simulink model "Controller_Exp"  (R2016a)
settings: Solver=ode4  StartTime=0.0  StopTime=Inf  FixedStep=Ts  RelTol=1e-3
undefined symbols (not defined in the file or in its folder): A_lpf_velocity, B1_lpf_velocity, B2_lpf_velocity, Calibration, commanded_u, GearOffsets, IMUTorsoOffsets, MedullaCommand, ResetDAQ, sample_time, TorsoCOMOffsets, Ts
libraries: xpcethercatlib x188, simulink x37, slrtlib x11, ControllerLibrary x2, dspswit3 x1
(part 1 of 4)
settings Model: TunableVars=GaitLibrary,GearOffsets,LegHipTorqueLimit,LimitSwHipAngle_ctrl,MedullaCommand,amp_ctrl,commanded_u,deltaStKA_ctrl,deltaSwHA_ctrl,deltaSwKA_ctrl,deltaSwLA_ctrl,floatDamper_ctrl,footPlacementHA_ctrl,footPlacementLA_ctrl,freq_ctrl,hold_ctrl,isTest_constantHips,isTest_doubleSupport,isTest_hipTracking,isTest_holdInAir,isTest_stopAndGo,jointPassivity_ctrl,joint_test_amp_ctrl,joint_test_freq_ctrl,joint_test_link_num_ctrl,joint_zero_ctrl,kd_ctrl,kd_hip_ctrl,kd_pitch,kd_roll,kd_sha,kd_sla,kd_stanceHip,kd_stanceKnee,kd_stanceLeg,kd_swingHip,kd_swingKnee,kd_swingLeg,kf_knee,kf_sha,kf_sla,kg_sha,kg_sla,ki_sha,ki_sla,kp_ctrl,kp_hip_ctrl,kp_pitch,kp_roll,kp_sha,kp_sla,kp_stanceHip,kp_stanceKnee,kp_stanceLeg,kp_swingHip,kp_swingKnee,kp_swingLeg,kp_yaw,leg_length,link_num_ctrl,ps3Axes,ps3Buttons,ps3Pov,regulate_velocity_ctrl,s_hold_ctrl,s_period_ctrl,stepTime,thres_hi,thres_lo,torso_com_offset,torso_control_ctrl,uHipGravity,zero_error_ctrl  TunableVarsStorageClass=Auto,Auto,Auto,Auto,Auto,Auto,Auto,Auto,Auto,Auto,Auto,Auto,Auto,Auto,Auto,Auto,Auto,Auto,Auto,Auto,Auto,Auto,Auto,Auto,Auto,Auto,Auto,Auto,Auto,Auto,Auto,Auto,Auto,Auto,Auto,Auto,Auto,Auto,Auto,Auto,Auto,Auto,Auto,Auto,Auto,Auto,Auto,Auto,Auto,Auto,Auto,Auto,Auto,Auto,Auto,Auto,Auto,Auto,Auto,Auto,Auto,Auto,Auto,Auto,Auto,Auto,Auto,Auto,Auto,Auto,Auto,Auto,Auto  TunableVarsTypeQualifier=,,,,,,,,,,,,,,,,,,,,,,,,,,,,,,,,,,,,,,,,,,,,,,,,,,,,,,,,,,,,,,,,,,,,,,,,  Creator=mvetsch  LastModifiedBy=gyk
settings SolverCC: EnableConcurrentExecution=on
settings DataIOCC: SaveFormat=Structure  SignalLoggingSaveFormat=ModelDataLogs  SaveState=on  SignalLoggingName=logsOut
settings OptimizationCC: BlockReduction=off  BooleanDataType=off  DefaultParameterBehavior=Inlined  OptimizeBlockIOStorage=off  BufferReuse=off  GlobalBufferReuse=off  ExpressionFolding=off  LocalBlockOutputs=off  InitFltsAndDblsToZero=on
settings DebuggingCC: SaveWithParameterizedLinksMsg=none  CheckExecutionContextPreStartOutputMsg=on  CheckExecutionContextRuntimeOutputMsg=on  SignalResolutionControl=TryResolveAllWithWarning  MultiTaskDSMMsg=warning  MultiTaskCondExecSysMsg=none
settings HardwareCC: ProdBitPerPointer=32  ProdLargestAtomicFloat=None  ProdWordSize=32  ProdLongLongMode=on  ProdHWDeviceType=Generic->32-bit x86 compatible
settings ModelReferenceCC: PropagateSignalLabelsOutOfModel=off
settings RTWCC: SystemTargetFile=slrt.tlc  TemplateMakefile=slrt_default_tmf  Description=Simulink Real-Time
settings SimulinkRealTimeCC: GeneratePreprocessorConditionals=Disable all  RL32LogBufSizeModifier=40000000  xPCisDownloadable=off
settings ConfigComp: CovModelRefEnable=Off  CovSFcnEnable=off

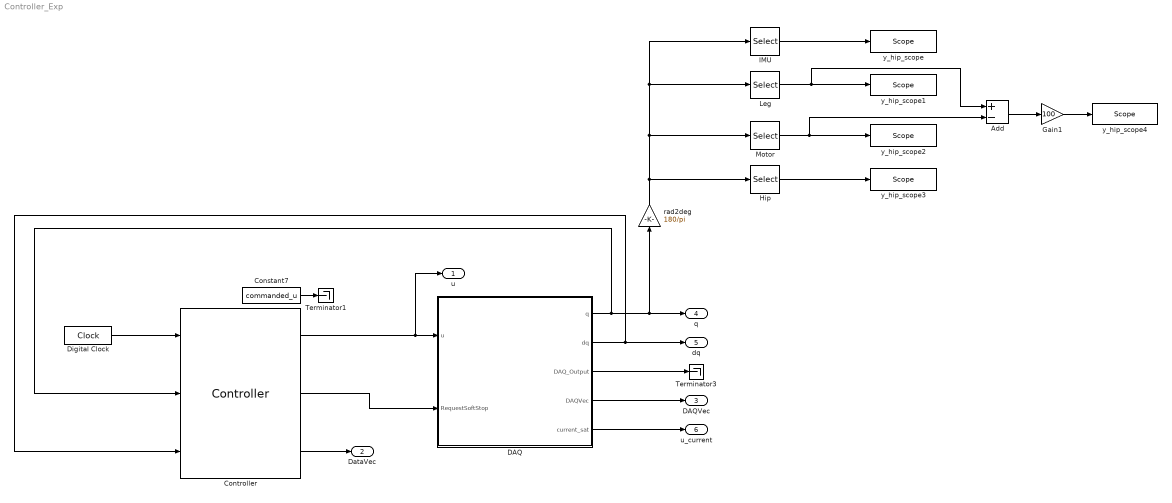
== system Controller_Exp ==
  Add : Sum  Inputs=+-
  Constant7 : Constant  Value=commanded_u
  Controller : ControllerLibrary/Controller
  DAQ : Subsystem
  Digital Clock : DigitalClock  SampleTime=Ts
  Gain1 : Gain  Gain=100
  Hip : Selector  InputPortWidth=13  IndexOptions=Index vector (dialog)  Indices=[10 13]  OutputSizes=1
  IMU : Selector  InputPortWidth=13  IndexOptions=Index vector (dialog)  Indices=[1 2 3]  OutputSizes=1
  Leg : Selector  InputPortWidth=13  IndexOptions=Index vector (dialog)  Indices=[4 5 6 7]  OutputSizes=1
  Motor : Selector  InputPortWidth=13  IndexOptions=Index vector (dialog)  Indices=[8 9 11 12]  OutputSizes=1
  Terminator1 : Terminator
  Terminator3 : Terminator
  rad2deg : Gain  Gain=180/pi
  y_hip_scope : slrtlib/Displays and Logging/Scope   scopeno=101  scopetype=Host  autostart=on  viewmode=Graphical redraw  formatstr='%15.6f'  grid=on  ylimits=[0,0]  nosamples=2500  noprepostsamples=0  interleave=1  triggermode=FreeRun  triggersignal=1  trigsignalfromport=off  triggerlevel=0.0  triggerslope=Either  triggerscope=1  triggersample=0  filename=data.dat  mode=Lazy  writesize=512  autorestart=off  dynamicfilemode=off  maxwritefilesize=512*1024^2
  y_hip_scope1 : slrtlib/Displays and Logging/Scope   scopeno=102  scopetype=Host  autostart=on  viewmode=Graphical redraw  formatstr='%15.6f'  grid=on  ylimits=[0,0]  nosamples=2500  noprepostsamples=0  interleave=1  triggermode=FreeRun  triggersignal=1  trigsignalfromport=off  triggerlevel=0.0  triggerslope=Either  triggerscope=1  triggersample=0  filename=data.dat  mode=Lazy  writesize=512  autorestart=off  dynamicfilemode=off  maxwritefilesize=512*1024^2
  y_hip_scope2 : slrtlib/Displays and Logging/Scope   scopeno=103  scopetype=Host  autostart=on  viewmode=Graphical redraw  formatstr='%15.6f'  grid=on  ylimits=[0,0]  nosamples=2500  noprepostsamples=0  interleave=1  triggermode=FreeRun  triggersignal=1  trigsignalfromport=off  triggerlevel=0.0  triggerslope=Either  triggerscope=1  triggersample=0  filename=data.dat  mode=Lazy  writesize=512  autorestart=off  dynamicfilemode=off  maxwritefilesize=512*1024^2
  y_hip_scope3 : slrtlib/Displays and Logging/Scope   scopeno=104  scopetype=Host  autostart=on  viewmode=Graphical redraw  formatstr='%15.6f'  grid=on  ylimits=[0,0]  nosamples=2500  noprepostsamples=0  interleave=1  triggermode=FreeRun  triggersignal=1  trigsignalfromport=off  triggerlevel=0.0  triggerslope=Either  triggerscope=1  triggersample=0  filename=data.dat  mode=Lazy  writesize=512  autorestart=off  dynamicfilemode=off  maxwritefilesize=512*1024^2
  y_hip_scope4 : slrtlib/Displays and Logging/Scope   scopeno=105  scopetype=Host  autostart=on  viewmode=Graphical redraw  formatstr='%15.6f'  grid=on  ylimits=[0,0]  nosamples=2500  noprepostsamples=0  interleave=1  triggermode=FreeRun  triggersignal=1  trigsignalfromport=off  triggerlevel=0.0  triggerslope=Either  triggerscope=1  triggersample=0  filename=data.dat  mode=Lazy  writesize=512  autorestart=off  dynamicfilemode=off  maxwritefilesize=512*1024^2
  u : Outport
  DataVec : Outport  Port=2
  DAQVec : Outport  Port=3
  q : Outport  Port=4
  dq : Outport  Port=5
  u_current : Outport  Port=6
  wires:
  IMU/1 -> y_hip_scope/1
  rad2deg/1 -> Motor/1, Leg/1, IMU/1, Hip/1
  Hip/1 -> y_hip_scope3/1
  Motor/1 -> y_hip_scope2/1, Add/2
  Leg/1 -> y_hip_scope1/1, Add/1
  Add/1 -> Gain1/1
  Digital Clock/1 -> Controller/1
  DAQ/4(DAQVec) -> DAQVec/1
  DAQ/1(q) -> Controller/2, q/1, rad2deg/1
  DAQ/2(dq) -> Controller/3, dq/1
  Controller/2 -> DAQ/2(RequestSoftStop)
  Controller/3 -> DataVec/1
  Gain1/1 -> y_hip_scope4/1
  DAQ/3(DAQ_Output) -> Terminator3/1
  Controller/1 -> u/1, DAQ/1(u)
  Constant7/1 -> Terminator1/1
  DAQ/5(current_sat) -> u_current/1

== system Controller_Exp/DAQ ==
  u : Inport
  RequestSoftStop : Inport  Port=2
  Bus Creator1 : BusCreator  Inputs='EncoderAngles','EncoderDerivs','MotorCurrentSafe','IMU_EulerAngles','IMU_EulerAnglesDerivs','MedullaCommandSafe','RotationMatrix','AbsTick','IncTick','ValidStates','SafetyState','IMU_Accel','IMU_AngularRate','EtherCATStatus','EncoderAnglesDirty','CurrentActual','FaultDetected','MedullaState','ErrorFlags','ElmoPosition'  OutDataTypeStr=Bus: DAQ_bus
  DAQ_sub : Subsystem
  DataBusSelector : BusSelector  OutputSignals=EncoderAngles,EncoderDerivs,MotorCurrentSafe,IMU_EulerAngles,IMU_EulerAnglesDerivs,MedullaCommandSafe,RotationMatrix,AbsTick,IncTick,ValidStates,SafetyState,IMU_Accel,IMU_AngularRate,EtherCATStatus,EncoderAnglesDirty,CurrentActual,FaultDetected,MedullaState,ErrorFlags,ElmoPosition
  DataVectorize : Concatenate  NumInputs=20
  q : Outport
  dq : Outport  Port=2
  DAQ_Output : Outport  Port=3
  DAQVec : Outport  Port=4
  current_sat : Outport  Port=5
  wires:
  DAQ_sub/1(q) -> q/1
  DAQ_sub/8(MedullaCommandSafe) -> Bus Creator1/6  "MedullaCommandSafe"
  DAQ_sub/3(EncoderAnglesClean) -> Bus Creator1/1  "EncoderAngles"
  DAQ_sub/11(IncTick) -> Bus Creator1/9  "IncTick"
  DAQ_sub/13(SafetyState) -> Bus Creator1/11  "SafetyState"
  DAQ_sub/7(EulerDerivsClean) -> Bus Creator1/5  "IMU_EulerAnglesDerivs"
  DAQ_sub/9(RotationMatrix) -> Bus Creator1/7  "RotationMatrix"
  DAQ_sub/4(EncoderDerivsClean) -> Bus Creator1/2  "EncoderDerivs"
  DAQ_sub/5(MotorCurrentSafe) -> Bus Creator1/3  "MotorCurrentSafe"
  DAQ_sub/12(ValidStates) -> Bus Creator1/10  "ValidStates"
  DAQ_sub/10(AbsTick) -> Bus Creator1/8  "AbsTick"
  DAQ_sub/6(EulerAnglesClean) -> Bus Creator1/4  "IMU_EulerAngles"
  DAQ_sub/14(IMU_Accel) -> Bus Creator1/12  "IMU_Accel"
  DAQ_sub/15(IMU_AngularRate) -> Bus Creator1/13  "IMU_AngularRate"
  DAQ_sub/2(dq) -> dq/1
  DataVectorize/1 -> DAQVec/1
  Bus Creator1/1 -> DataBusSelector/1, DAQ_Output/1
  DataBusSelector/6 -> DataVectorize/6  "<MedullaCommandSafe>"
  DataBusSelector/7 -> DataVectorize/7  "<RotationMatrix>"
  DataBusSelector/9 -> DataVectorize/9  "<IncTick>"
  DataBusSelector/12 -> DataVectorize/12  "<IMU_Accel>"
  DataBusSelector/10 -> DataVectorize/10  "<ValidStates>"
  DataBusSelector/11 -> DataVectorize/11  "<SafetyState>"
  DataBusSelector/13 -> DataVectorize/13  "<IMU_AngularRate>"
  DataBusSelector/8 -> DataVectorize/8  "<AbsTick>"
  u/1 -> DAQ_sub/1(u)
  RequestSoftStop/1 -> DAQ_sub/2(RequestSoftStop)
  DAQ_sub/16(EtherCATStatus) -> Bus Creator1/14  "EtherCATStatus"
  DataBusSelector/14 -> DataVectorize/14  "<EtherCATStatus>"
  DAQ_sub/17(EncoderAnglesDirty) -> Bus Creator1/15  "EncoderAnglesDirty"
  DataBusSelector/15 -> DataVectorize/15  "<EncoderAnglesDirty>"
  DAQ_sub/18(CurrentActual) -> Bus Creator1/16  "CurrentActual"
  DAQ_sub/19(FaultDetected) -> Bus Creator1/17  "FaultDetected"
  DataBusSelector/16 -> DataVectorize/16  "<CurrentActual>"
  DataBusSelector/17 -> DataVectorize/17  "<FaultDetected>"
  DAQ_sub/20(MedullaState) -> Bus Creator1/18  "MedullaState"
  DAQ_sub/21(ErrorFlags) -> Bus Creator1/19  "ErrorFlags"
  DataBusSelector/18 -> DataVectorize/18  "<MedullaState>"
  DataBusSelector/19 -> DataVectorize/19  "<ErrorFlags>"
  DataBusSelector/1 -> DataVectorize/1  "<EncoderAngles>"
  DataBusSelector/2 -> DataVectorize/2  "<EncoderDerivs>"
  DataBusSelector/3 -> DataVectorize/3  "<MotorCurrentSafe>"
  DataBusSelector/4 -> DataVectorize/4  "<IMU_EulerAngles>"
  DataBusSelector/5 -> DataVectorize/5  "<IMU_EulerAnglesDerivs>"
  DAQ_sub/22(ElmoPosition) -> Bus Creator1/20  "ElmoPosition"
  DataBusSelector/20 -> DataVectorize/20  "<ElmoPosition>"
  DAQ_sub/23(current_sat) -> current_sat/1

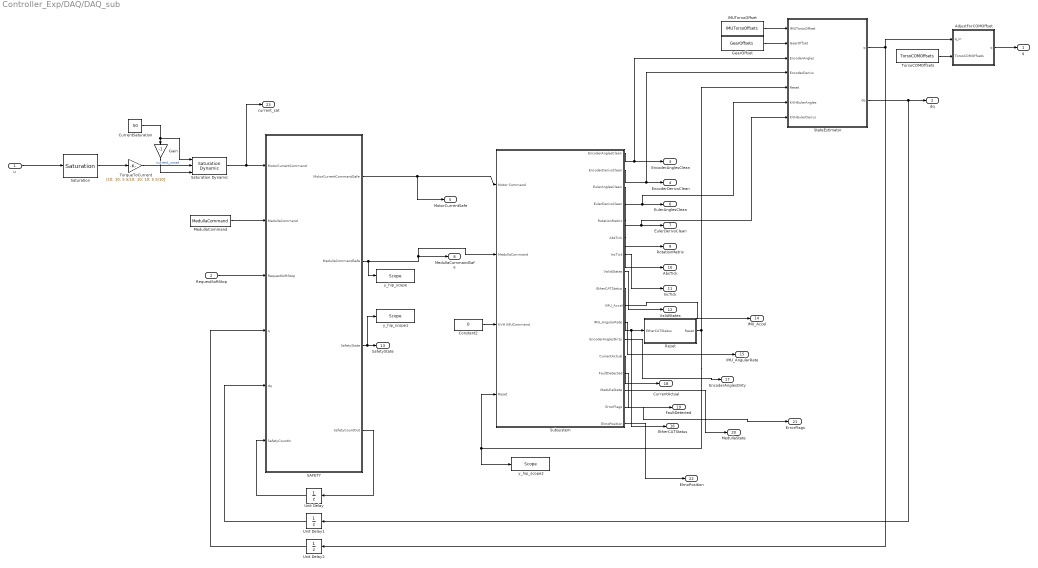
== system Controller_Exp/DAQ/DAQ_sub ==
  u : Inport
  RequestSoftStop : Inport  Port=2
  AdjustForCOMOffset : MATLAB Function  TreatAsAtomicUnit=on
  Constant2 : Constant  Value=0
  CurrentSaturation : Constant  Value=50
  Gain : Gain  Gain=-1
  GearOffset : Constant  Value=GearOffsets
  IMUTorsoOffset : Constant  Value=IMUTorsoOffsets
  MedullaCommand : Constant  Value=MedullaCommand
  Reset : Subsystem
  SAFETY : MATLAB Function  TreatAsAtomicUnit=on
  Saturation : ControllerLibrary/Controller/Saturation
  Saturation Dynamic : simulink/Discontinuities/Saturation Dynamic  OutMin=[]  OutMax=[]  OutDataTypeStr=Inherit: Same as second input  OutDataType=fixdt(1, 16)  OutScaling=2^-10  DoSatur=off
  StateEstimator : Subsystem
  Subsystem : Subsystem
  TorqueToCurrent : Gain  Gain=[10; 10; 5.5/10; 10; 10; 5.5/10]
  TorsoCOMOffsets : Constant  Value=TorsoCOMOffsets
  Unit Delay : UnitDelay  SampleTime=-1
  Unit Delay1 : UnitDelay  SampleTime=-1
  Unit Delay2 : UnitDelay  SampleTime=-1
  y_hip_scope : slrtlib/Displays and Logging/Scope   scopeno=106  scopetype=Host  autostart=on  viewmode=Graphical redraw  formatstr='%15.6f'  grid=on  ylimits=[0,0]  nosamples=2500  noprepostsamples=0  interleave=1  triggermode=FreeRun  triggersignal=1  trigsignalfromport=off  triggerlevel=0.0  triggerslope=Either  triggerscope=1  triggersample=0  filename=data.dat  mode=Lazy  writesize=512  autorestart=off  dynamicfilemode=off  maxwritefilesize=512*1024^2
  y_hip_scope1 : slrtlib/Displays and Logging/Scope   scopeno=107  scopetype=Host  autostart=on  viewmode=Graphical redraw  formatstr='%15.6f'  grid=on  ylimits=[0,0]  nosamples=2500  noprepostsamples=0  interleave=1  triggermode=FreeRun  triggersignal=1  trigsignalfromport=off  triggerlevel=0.0  triggerslope=Either  triggerscope=1  triggersample=0  filename=data.dat  mode=Lazy  writesize=512  autorestart=off  dynamicfilemode=off  maxwritefilesize=512*1024^2
  y_hip_scope2 : slrtlib/Displays and Logging/Scope   scopeno=108  scopetype=Host  autostart=on  viewmode=Graphical redraw  formatstr='%15.6f'  grid=on  ylimits=[0,0]  nosamples=2500  noprepostsamples=0  interleave=1  triggermode=FreeRun  triggersignal=1  trigsignalfromport=off  triggerlevel=0.0  triggerslope=Either  triggerscope=1  triggersample=0  filename=data.dat  mode=Lazy  writesize=512  autorestart=off  dynamicfilemode=off  maxwritefilesize=512*1024^2
  q : Outport
  dq : Outport  Port=2
  EncoderAnglesClean : Outport  Port=3
  EncoderDerivsClean : Outport  Port=4
  MotorCurrentSafe : Outport  Port=5
  EulerAnglesClean : Outport  Port=6
  EulerDerivsClean : Outport  Port=7
  MedullaCommandSafe : Outport  Port=8
  RotationMatrix : Outport  Port=9
  AbsTick : Outport  Port=10
  IncTick : Outport  Port=11
  ValidStates : Outport  Port=12
  SafetyState : Outport  Port=13
  IMU_Accel : Outport  Port=14
  IMU_AngularRate : Outport  Port=15
  EtherCATStatus : Outport  Port=16
  EncoderAnglesDirty : Outport  Port=17
  CurrentActual : Outport  Port=18
  FaultDetected : Outport  Port=19
  MedullaState : Outport  Port=20
  ErrorFlags : Outport  Port=21
  ElmoPosition : Outport  Port=22
  current_sat : Outport  Port=23
  wires:
  TorqueToCurrent/1 -> Saturation Dynamic/2  "current_unsat"
  Gain/1 -> Saturation Dynamic/3
  Unit Delay/1 -> SAFETY/6(SafetyCountIn)
  CurrentSaturation/1 -> Saturation Dynamic/1, Gain/1
  Unit Delay2/1 -> SAFETY/4(q)
  MedullaCommand/1 -> SAFETY/2(MedullaCommand)
  StateEstimator/2(dq) -> dq/1, Unit Delay1/1
  Unit Delay1/1 -> SAFETY/5(dq)
  SAFETY/4(SafetyCountOut) -> Unit Delay/1
  SAFETY/3(SafetyState) -> y_hip_scope1/1, SafetyState/1
  SAFETY/2(MedullaCommandSafe) -> y_hip_scope/1, MedullaCommandSafe/1, Subsystem/2(MedullaCommand)
  Subsystem/4(EulerDerivsClean) -> EulerDerivsClean/1, StateEstimator/7(KVHEulerDerivs)
  Reset/1(Reset) -> y_hip_scope2/1, Subsystem/4(Reset), StateEstimator/5(Reset)
  Constant2/1 -> Subsystem/3(KVH IMUCommand)
  Subsystem/6(AbsTick) -> AbsTick/1
  Subsystem/7(IncTick) -> IncTick/1
  Subsystem/8(ValidStates) -> ValidStates/1
  Subsystem/5(RotationMatrix) -> RotationMatrix/1
  GearOffset/1 -> StateEstimator/2(GearOffset)
  Subsystem/3(EulerAnglesClean) -> StateEstimator/6(KVHEulerAngles), EulerAnglesClean/1
  Subsystem/1(EncoderAnglesClean) -> EncoderAnglesClean/1, StateEstimator/3(EncoderAngles)
  Subsystem/2(EncoderDerivsClean) -> EncoderDerivsClean/1, StateEstimator/4(EncoderDerivs)
  IMUTorsoOffset/1 -> StateEstimator/1(IMUTorsoOffset)
  SAFETY/1(MotorCurrentCommandSafe) -> MotorCurrentSafe/1, Subsystem/1(Motor Command)
  TorsoCOMOffsets/1 -> AdjustForCOMOffset/2(TorsoCOMOffsets)
  AdjustForCOMOffset/1(q) -> q/1
  StateEstimator/1(q) -> AdjustForCOMOffset/1(q_in), Unit Delay2/1
  RequestSoftStop/1 -> SAFETY/3(RequestSoftStop)
  Subsystem/10(IMU_Accel) -> IMU_Accel/1
  Subsystem/11(IMU_AngularRate) -> IMU_AngularRate/1
  Subsystem/9(EtherCATStatus) -> EtherCATStatus/1, Reset/1(EtherCATStatus)
  Subsystem/12(EncoderAnglesDirty) -> EncoderAnglesDirty/1
  Subsystem/13(CurrentActual) -> CurrentActual/1
  Subsystem/14(FaultDetected) -> FaultDetected/1
  Subsystem/15(MedullaState) -> MedullaState/1
  Subsystem/16(ErrorFlags) -> ErrorFlags/1
  Subsystem/17(ElmoPosition) -> ElmoPosition/1
  u/1 -> Saturation/1
  Saturation/1 -> TorqueToCurrent/1
  Saturation Dynamic/1 -> current_sat/1, SAFETY/1(MotorCurrentCommand)

== system Controller_Exp/DAQ/DAQ_sub/Reset ==
  note: EtherCATStatus is a vector of six elements:
      | [ErrVal MasterState DCErrVal MasterToNetworkClkDiff
      | DCInitState NetworkToSlaveClkDiff]
      | Here we just check that MasterState==8 (Operational state),
      | the DC is started, and that there is no DC error.
  EtherCATStatus : Inport
  Compare To Constant : simulink/Logic and Bit Operations/Compare To Constant  relop=<=  const=12.0  OutDataTypeStr=boolean
  Compare To Constant1 : simulink/Logic and Bit Operations/Compare To Constant  relop=~=  const=8  OutDataTypeStr=boolean
  Digital Clock : DigitalClock  SampleTime=Ts
  Logical Operator : Logic  Operator=OR  OutDataTypeStr=boolean
  Logical Operator1 : Logic  Operator=OR  OutDataTypeStr=boolean
  Logical Operator2 : Logic  OutDataTypeStr=boolean
  ResetDAQ1 : Constant  Value=ResetDAQ  OutDataTypeStr=boolean
  Selector : Selector  IndexMode=Zero-based  InputPortWidth=6  IndexOptions=Index vector (dialog)  Indices=1  OutputSizes=1
  Unit Delay : UnitDelay  InitialCondition=1  SampleTime=-1
  Reset : Outport
  wires:
  Logical Operator2/1 -> Unit Delay/1
  Unit Delay/1 -> Logical Operator1/2, Logical Operator2/2
  Logical Operator/1 -> Logical Operator2/1
  Logical Operator1/1 -> Reset/1
  ResetDAQ1/1 -> Logical Operator1/1
  Compare To Constant/1 -> Logical Operator/1
  Digital Clock/1 -> Compare To Constant/1
  Compare To Constant1/1 -> Logical Operator/2
  EtherCATStatus/1 -> Selector/1
  Selector/1 -> Compare To Constant1/1

== system Controller_Exp/DAQ/DAQ_sub/StateEstimator ==
  IMUTorsoOffset : Inport
  GearOffset : Inport  Port=2
  EncoderAngles : Inport  Port=3
  EncoderDerivs : Inport  Port=4
  Reset : Inport  Port=5
  KVHEulerAngles : Inport  Port=6
  KVHEulerDerivs : Inport  Port=7
  GeneralizedCoordinates : MATLAB Function  TreatAsAtomicUnit=on
  UseIMU : Constant
  UseMotorIncEncoders : Constant  Value=0
  q : Outport
  dq : Outport  Port=2
  wires:
  KVHEulerDerivs/1 -> GeneralizedCoordinates/4(IMUVelocities)
  KVHEulerAngles/1 -> GeneralizedCoordinates/3(IMUAngles)
  EncoderDerivs/1 -> GeneralizedCoordinates/2(EncoderVelocities)
  EncoderAngles/1 -> GeneralizedCoordinates/1(EncoderAngles)
  Reset/1 -> GeneralizedCoordinates/9(Reset)
  GeneralizedCoordinates/1(q_clean) -> q/1
  GeneralizedCoordinates/2(dq_clean) -> dq/1
  IMUTorsoOffset/1 -> GeneralizedCoordinates/7(IMUTorsoOffset)
  UseMotorIncEncoders/1 -> GeneralizedCoordinates/5(UseMotorIncEncoders)
  GearOffset/1 -> GeneralizedCoordinates/8(GearOffset)
  UseIMU/1 -> GeneralizedCoordinates/6(UseIMU)

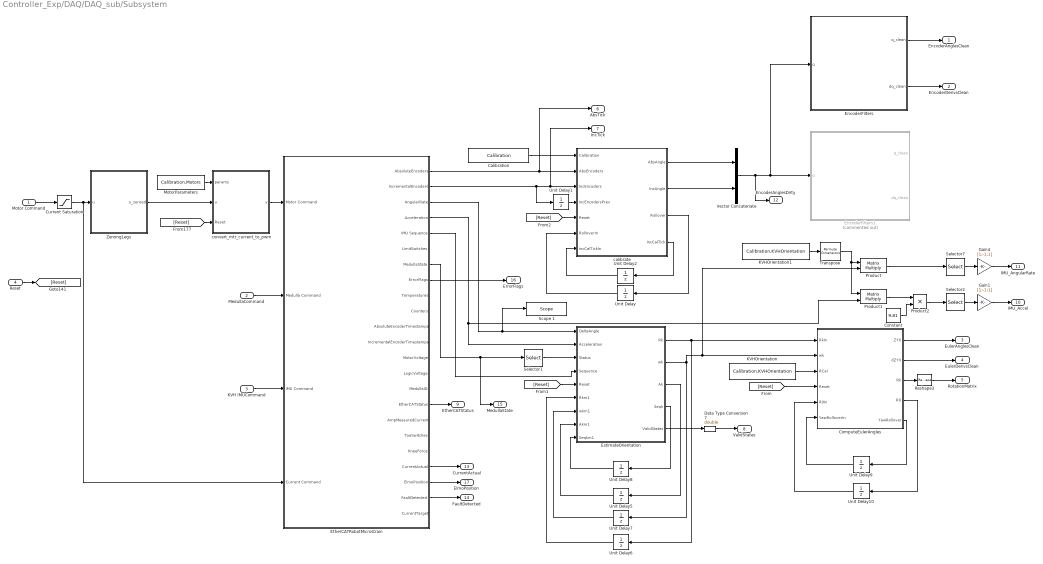
== system Controller_Exp/DAQ/DAQ_sub/Subsystem ==
  Motor Command : Inport
  MedullaCommand : Inport  Port=2
  KVH IMUCommand : Inport  Port=3
  Reset : Inport  Port=4
  Calibration : Constant  Value=Calibration  OutDataTypeStr=Bus: RobotCalibrationBus
  ComputeEulerAngles : MATLAB Function  TreatAsAtomicUnit=on
  Constant : Constant  Value=9.81
  Current Saturation : Saturate  UpperLimit=50  LowerLimit=-50
  Data Type Conversion7 : DataTypeConversion  OutDataTypeStr=double
  EncoderFilters : Subsystem
  EncoderFilters1 : Subsystem  Commented=on  TreatAsAtomicUnit=on
  EstimateOrientation : MATLAB Function  TreatAsAtomicUnit=on
  EtherCATRobotMicrostrain : Subsystem
  Gain1 : Gain  Gain=[1;-1;1]
  Gain4 : Gain  Gain=[1;-1;1]
  KVHOrientation : Constant  Value=Calibration.KVHOrientation
  KVHOrientation1 : Constant  Value=Calibration.KVHOrientation
  MotorParameters : Constant  Value=Calibration.Motors
  Product : Product  Multiplication=Matrix(*)
  Product1 : Product  Multiplication=Matrix(*)
  Product2 : Product
  Reshape3 : Reshape
  Scope 1 : slrtlib/Displays and Logging/Scope   scopeno=109  scopetype=Host  autostart=on  viewmode=Graphical redraw  formatstr='%15.6f'  grid=on  ylimits=[0,0]  nosamples=2500  noprepostsamples=0  interleave=1  triggermode=FreeRun  triggersignal=1  trigsignalfromport=off  triggerlevel=0.0  triggerslope=Either  triggerscope=1  triggersample=0  filename=data.dat  mode=Lazy  writesize=512  autorestart=off  dynamicfilemode=off  maxwritefilesize=512*1024^2
  Selector1 : Selector  IndexMode=Zero-based  InputPortWidth=7  IndexOptions=Index vector (dialog)  Indices=[6]  OutputSizes=1
  Selector2 : Selector  InputPortWidth=3  IndexOptions=Index vector (dialog)  Indices=[2,1,3]  OutputSizes=1
  Selector7 : Selector  InputPortWidth=3  IndexOptions=Index vector (dialog)  Indices=[2,1,3]  OutputSizes=1
  Transpose : PermuteDimensions
  Unit Delay : UnitDelay  InitialCondition=zeros(9,1)  SampleTime=-1
  Unit Delay1 : UnitDelay  SampleTime=-1
  Unit Delay10 : UnitDelay  InitialCondition=zeros(3,3)  SampleTime=-1
  Unit Delay2 : UnitDelay  InitialCondition=zeros(6,1)  SampleTime=-1
  Unit Delay5 : UnitDelay  InitialCondition=[0; 0; 0]  SampleTime=-1
  Unit Delay6 : UnitDelay  InitialCondition=zeros(3,3)  SampleTime=-1
  Unit Delay7 : UnitDelay  InitialCondition=[0; 0; 0]  SampleTime=-1
  Unit Delay8 : UnitDelay  SampleTime=-1
  Unit Delay9 : UnitDelay  InitialCondition=[0; 0]  SampleTime=-1
  Vector Concatenate : Concatenate
  ZeroingLegs : MATLAB Function  TreatAsAtomicUnit=on
  calibrate : MATLAB Function  TreatAsAtomicUnit=on
  convert_mtr_current_to_pwm : MATLAB Function  TreatAsAtomicUnit=on
  EncoderAnglesClean : Outport
  EncoderDerivsClean : Outport  Port=2
  EulerAnglesClean : Outport  Port=3
  EulerDerivsClean : Outport  Port=4
  RotationMatrix : Outport  Port=5
  AbsTick : Outport  Port=6
  IncTick : Outport  Port=7
  ValidStates : Outport  Port=8
  EtherCATStatus : Outport  Port=9
  IMU_Accel : Outport  Port=10
  IMU_AngularRate : Outport  Port=11
  EncoderAnglesDirty : Outport  Port=12
  CurrentActual : Outport  Port=13
  FaultDetected : Outport  Port=14
  MedullaState : Outport  Port=15
  ErrorFlags : Outport  Port=16
  ElmoPosition : Outport  Port=17
  wires:
  Motor Command/1 -> Current Saturation/1
  EncoderFilters/2(dq_clean) -> EncoderDerivsClean/1
  Unit Delay6/1 -> EstimateOrientation/6(Rkm1)
  EtherCATRobotMicrostrain/2(IncrementalEncoders) -> Unit Delay1/1, IncTick/1, calibrate/3(IncEncoders)
  Unit Delay8/1 -> EstimateOrientation/9(Seqkm1)
  calibrate/4(IncCalTick) -> Unit Delay2/1
  EtherCATRobotMicrostrain/1(AbsoluteEncoders) -> AbsTick/1, calibrate/2(AbsEncoders)
  Unit Delay/1 -> calibrate/6(RolloverIn)
  Unit Delay2/1 -> calibrate/7(IncCalTickIn)
  Unit Delay5/1 -> EstimateOrientation/8(Akm1)
  EstimateOrientation/3(Ak) -> Unit Delay5/1
  MedullaCommand/1 -> EtherCATRobotMicrostrain/2(Medulla Command)
  [Reset] -> calibrate/5(Reset)
  calibrate/2(IncAngle) -> Vector Concatenate/2
  convert_mtr_current_to_pwm/1(y) -> EtherCATRobotMicrostrain/1(Motor Command)
  Unit Delay1/1 -> calibrate/4(IncEncodersPrev)
  calibrate/1(AbsAngle) -> Vector Concatenate/1
  calibrate/3(Rollover) -> Unit Delay/1
  Calibration/1 -> calibrate/1(Calibration)
  Unit Delay7/1 -> EstimateOrientation/7(wkm1)
  EstimateOrientation/4(Seqk) -> Unit Delay8/1
  KVH IMUCommand/1 -> EtherCATRobotMicrostrain/3(IMU Command)
  EncoderFilters/1(q_clean) -> EncoderAnglesClean/1
  Unit Delay9/1 -> ComputeEulerAngles/6(YawRolloverIn)
  EtherCATRobotMicrostrain/5(IMU Sequence) -> EstimateOrientation/4(Sequence)
  ComputeEulerAngles/4(R0) -> Unit Delay10/1
  EstimateOrientation/1(Rk) -> Unit Delay6/1, ComputeEulerAngles/1(RkIn)
  ComputeEulerAngles/1(ZYX) -> EulerAnglesClean/1
  EstimateOrientation/5(ValidStates) -> Data Type Conversion7/1
  Selector1/1 -> EstimateOrientation/3(Status)
  ComputeEulerAngles/2(dZYX) -> EulerDerivsClean/1
  [Reset] -> ComputeEulerAngles/4(Reset)
  ComputeEulerAngles/3(Rk) -> Reshape3/1
  [Reset] -> EstimateOrientation/5(Reset)
  Data Type Conversion7/1 -> ValidStates/1
  ComputeEulerAngles/5(YawRollover) -> Unit Delay9/1
  KVHOrientation/1 -> ComputeEulerAngles/3(RCal)
  Reshape3/1 -> RotationMatrix/1
  EtherCATRobotMicrostrain/4(Acceleration) -> EstimateOrientation/2(Acceleration), Product1/2
  EtherCATRobotMicrostrain/3(AngularRate) -> Scope 1/1, EstimateOrientation/1(DeltaAngle)
  EtherCATRobotMicrostrain/7(MedullaState) -> MedullaState/1, Selector1/1
  Unit Delay10/1 -> ComputeEulerAngles/5(R0In)
  EstimateOrientation/2(wk) -> Unit Delay7/1, Product/2, ComputeEulerAngles/2(wk)
  Reset/1 -> [Reset]
  ZeroingLegs/1(u_zeroed) -> convert_mtr_current_to_pwm/2(u)
  Current Saturation/1 -> EtherCATRobotMicrostrain/4(Current Command), ZeroingLegs/1(u)
  MotorParameters/1 -> convert_mtr_current_to_pwm/1(params)
  [Reset] -> convert_mtr_current_to_pwm/3(Reset)
  EtherCATRobotMicrostrain/16(EtherCATStatus) -> EtherCATStatus/1
  KVHOrientation1/1 -> Transpose/1
  Transpose/1 -> Product1/1, Product/1
  Product1/1 -> Product2/1
  Constant/1 -> Product2/2
  Vector Concatenate/1 -> EncoderAnglesDirty/1, EncoderFilters/1(q), EncoderFilters1/1(q)
  EtherCATRobotMicrostrain/20(CurrentActual) -> CurrentActual/1
  EtherCATRobotMicrostrain/22(FaultDetected) -> FaultDetected/1
  EtherCATRobotMicrostrain/8(ErrorFlags) -> ErrorFlags/1
  Selector7/1 -> Gain4/1
  Product/1 -> Selector7/1
  Gain4/1 -> IMU_AngularRate/1
  Selector2/1 -> Gain1/1
  Gain1/1 -> IMU_Accel/1
  Product2/1 -> Selector2/1
  EtherCATRobotMicrostrain/21(ElmoPosition) -> ElmoPosition/1

== system Controller_Exp/DAQ/DAQ_sub/Subsystem/EncoderFilters ==
  q : Inport  Partition=on  PartitionDimension=1  PartitionWidth=1
  Filter : Subsystem
  For Each : ForEach  DisableCoverage=on  IndexMode=One-based
  Terminator7 : Terminator
  q_clean : Outport  ConcatenationDimension=1
  dq_clean : Outport  Port=2  ConcatenationDimension=1
  wires:
  q/1 -> Filter/1(q)
  Filter/1(q_clean) -> q_clean/1
  Filter/3(dq_clean_original) -> Terminator7/1
  Filter/2(dq_clean) -> dq_clean/1

== system Controller_Exp/DAQ/DAQ_sub/Subsystem/EncoderFilters1 ==
  q : Inport  Partition=on  PartitionDimension=1  PartitionWidth=1
  CheckAndFilterEncoder : Subsystem
  For Each : ForEach  DisableCoverage=on  IndexMode=One-based
  Terminator7 : Terminator
  q_clean : Outport  ConcatenationDimension=1
  dq_clean : Outport  Port=2  ConcatenationDimension=1
  wires:
  CheckAndFilterEncoder/3(dq_clean_origin) -> Terminator7/1
  q/1 -> CheckAndFilterEncoder/1(q_daq)
  CheckAndFilterEncoder/1(q_clean) -> q_clean/1
  CheckAndFilterEncoder/2(dq_clean) -> dq_clean/1

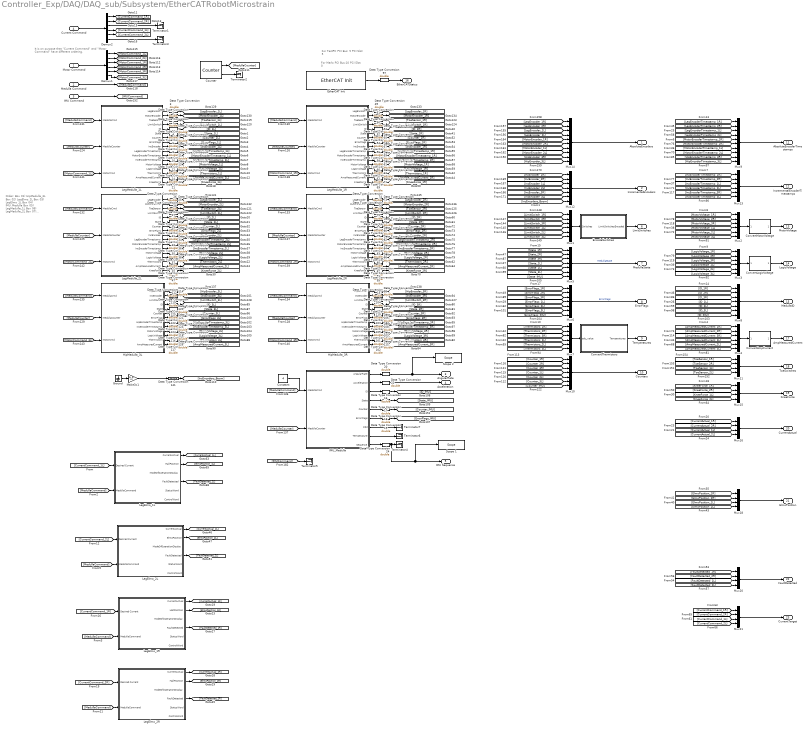
== system Controller_Exp/DAQ/DAQ_sub/Subsystem/EtherCATRobotMicrostrain ==
  note: Order:
      | Box 01) HipMedulla_3L
      | Box 02) LegElmo_2L
      | Box 03) LegElmo_1L
      | Box 04) IMU_Medulla
      | Box 05) LegMedulla_1L
      | Box 06) LegMedulla_2L
      | Box 07) LegMedulla_2R
      | Box 08) LegMedulla_1R
      | Box 09) LegElmo_2R
      | Box 10) LegElmo_1R
      | Box 11) HipMedulla_3R
  note: For TestPC
      | PCI Bus: 5 PCI Slot: 5
  note: For Marlo
      | PCI Bus:10 PCI Slot: 0
  note: It is on purpose that "Current Command"
      | and "Motor Command" have different ordering.
  Motor Command : Inport
  Medulla Command : Inport  Port=2
  IMU Command : Inport  Port=3
  Current Command : Inport  Port=4
  Constant : Constant  Value=4
  ConvertAmpCurrent : MATLAB Function  TreatAsAtomicUnit=on
  ConvertLogicVoltage : MATLAB Function  TreatAsAtomicUnit=on
  ConvertMotorVoltage : MATLAB Function  TreatAsAtomicUnit=on
  ConvertThermistors : MATLAB Function  TreatAsAtomicUnit=on
  Counter : dspswit3/Counter  Direction=Up  CountEvent=Free running  CounterSize=User defined  MaxCount=65535  InitialCount=0  Output=Count and Hit  HitValue=32  ResetInput=off  SamplesPerFrame=1  Ts=Ts  CntDtype=double  HitDtype=Logical
  Data Type Conversion{1..39,45,47,49..63,69,71,73..87,93,95,97..98,101..112,114,116..126,141,157} (103 alike) : DataTypeConversion  OutDataTypeStr=double
  Demux1 : Demux  Outputs=6
  Demux2 : Demux  Outputs=6
  EncodeSwitches : MATLAB Function  TreatAsAtomicUnit=on
  "EtherCAT Init " : xpcethercatlib/EtherCAT Init   Priority=0  config_file=D:\Graduate\robots\GitHub\3D_Marlo_Yukai\MARLO experiment\simulation\compliant_simulator\DAQ\500us\EtherCat_Files\MARLO-2.0_All-1ms.eni.xml  device_id=3  pci_bus=2  pci_slot=0  dctuning=0  enaDebug=off  enaDC=on  errLink=off  masterDbg=off  stateChgDbg=off  baseClock=off  masterCfg=off  logFile='c:\dbglog.txt'  sample_time=0.001000
  Ground : Ground
  HipMedulla_3L : Subsystem
  HipMedulla_3R : Subsystem
  IMU_Medulla : Subsystem
  LegElmo_1L : Subsystem
  LegElmo_1R : Subsystem
  LegElmo_2L : Subsystem
  LegElmo_2R : Subsystem
  LegMedulla_1L : Subsystem
  LegMedulla_1R : Subsystem
  LegMedulla_2L : Subsystem
  LegMedulla_2R : Subsystem
  Make3x1 : Gain  Gain=[0; 0; 0]
  Mux{1..4,7,13} (6 alike) : Mux  Inputs=6
  Mux{5..6,8,10,12} (5 alike) : Mux  Inputs=7
  Mux{11,15..16,18,20..21} (6 alike) : Mux
  Mux14 : Mux  Inputs=10
  Mux9 : Mux  Inputs=10
  Scope 1 : slrtlib/Displays and Logging/Scope   scopeno=110  scopetype=Host  autostart=on  viewmode=Graphical redraw  formatstr='%15.6f'  grid=on  ylimits=[0,0]  nosamples=2500  noprepostsamples=0  interleave=1  triggermode=FreeRun  triggersignal=1  trigsignalfromport=off  triggerlevel=0.0  triggerslope=Either  triggerscope=1  triggersample=0  filename=data.dat  mode=Lazy  writesize=512  autorestart=off  dynamicfilemode=off  maxwritefilesize=512*1024^2
  Scope 2 : slrtlib/Displays and Logging/Scope   scopeno=111  scopetype=Host  autostart=on  viewmode=Graphical redraw  formatstr='%15.6f'  grid=on  ylimits=[0,0]  nosamples=2500  noprepostsamples=0  interleave=1  triggermode=FreeRun  triggersignal=1  trigsignalfromport=off  triggerlevel=0.0  triggerslope=Either  triggerscope=1  triggersample=0  filename=data.dat  mode=Lazy  writesize=512  autorestart=off  dynamicfilemode=off  maxwritefilesize=512*1024^2
  Terminator{1..7} (7 alike) : Terminator
  AbsoluteEncoders : Outport
  IncrementalEncoders : Outport  Port=2
  AngularRate : Outport  Port=3
  Acceleration : Outport  Port=4
  IMU Sequence : Outport  Port=5
  LimitSwitches : Outport  Port=6
  MedullaState : Outport  Port=7
  ErrorFlags : Outport  Port=8
  Temperatures : Outport  Port=9
  Counters : Outport  Port=10
  AbsoluteEncoderTimestamps : Outport  Port=11
  IncrementalEncoderTimestamps : Outport  Port=12
  MotorVoltage : Outport  Port=13
  LogicVoltage : Outport  Port=14
  MedullaID : Outport  Port=15
  EtherCATStatus : Outport  Port=16
  AmpMeasuredCurrent : Outport  Port=17
  ToeSwitches : Outport  Port=18
  KneeForce : Outport  Port=19
  CurrentActual : Outport  Port=20
  ElmoPosition : Outport  Port=21
  FaultDetected : Outport  Port=22
  CurrentTarget : Outport  Port=23
  wires:
  Data Type Conversion22/1 -> Acceleration/1
  [CurrentCommand_2L] -> Mux21/4
  [CurrentCommand_1L] -> Mux21/3
  [CurrentCommand_2R] -> Mux21/2
  [CurrentCommand_1R] -> Mux21/1
  Mux21/1 -> CurrentTarget/1
  Demux2/6 -> Terminator3/1
  Demux2/4 -> [CurrentCommand_1L]
  Demux2/3 -> Terminator1/1
  Demux2/2 -> [CurrentCommand_2R]
  Demux2/5 -> [CurrentCommand_2L]
  Demux2/1 -> [CurrentCommand_1R]
  LegElmo_1L/4(FaultDetected) -> [FaultDetected_1L]
  LegElmo_1L/2(HallPosition) -> [ElmoPosition_1L]
  LegElmo_1L/1(CurrentActual) -> [CurrentActual_1L]
  LegElmo_2L/4(FaultDetected) -> [FaultDetected_2L]
  LegElmo_2L/2(ElmoPosition) -> [ElmoPosition_2L]
  LegElmo_2L/1(CurrentActual) -> [CurrentActual_2L]
  LegElmo_2R/4(FaultDetected) -> [FaultDetected_2R]
  LegElmo_2R/2(HallPosition) -> [ElmoPosition_2R]
  LegElmo_2R/1(CurrentActual) -> [CurrentActual_2R]
  LegElmo_1R/4(FaultDetected) -> [FaultDetected_1R]
  LegElmo_1R/2(HallPosition) -> [ElmoPosition_1R]
  LegElmo_1R/1(CurrentActual) -> [CurrentActual_1R]
  [FaultDetected_2L] -> Mux20/4
  [FaultDetected_1L] -> Mux20/3
  [FaultDetected_2R] -> Mux20/2
  [FaultDetected_1R] -> Mux20/1
  Mux20/1 -> FaultDetected/1
  [ElmoPosition_2L] -> Mux18/4
  [ElmoPosition_1L] -> Mux18/3
  [ElmoPosition_2R] -> Mux18/2
  [ElmoPosition_1R] -> Mux18/1
  Mux18/1 -> ElmoPosition/1
  [CurrentActual_2L] -> Mux16/4
  [CurrentActual_1L] -> Mux16/3
  [CurrentActual_2R] -> Mux16/2
  [CurrentActual_1R] -> Mux16/1
  Mux16/1 -> CurrentActual/1
  [CurrentCommand_2R] -> LegElmo_2R/1(Desired Current)
  [CurrentCommand_1R] -> LegElmo_1R/1(Desired Current)
  [CurrentCommand_2L] -> LegElmo_2L/1(Desired Current)
  [CurrentCommand_1L] -> LegElmo_1L/1(Desired Current)
  Current Command/1 -> Demux2/1
  [MedullaCommand] -> LegElmo_2R/2(MedullaCommand)
  [MedullaCommand] -> LegElmo_2L/2(MedullaCommand)
  [MedullaCommand] -> LegElmo_1R/2(MedullaCommand)
  [MedullaCommand] -> LegElmo_1L/2(MedullaCommand)
  Data Type Conversion19/1 -> [ErrorFlags_IMU]
  Data Type Conversion18/1 -> [Counter_IMU]
  Data Type Conversion17/1 -> [State_IMU]
  Data Type Conversion16/1 -> [ID_IMU]
  [IncEncoders_Boom] -> Mux12/7
  Make3x1/1 -> Data Type Conversion141/1
  Ground/1 -> Make3x1/1
  [KneeForce_2L] -> Mux15/4
  [KneeForce_1L] -> Mux15/3
  [KneeForce_2R] -> Mux15/2
  [KneeForce_1R] -> Mux15/1
  Mux15/1 -> KneeForce/1
  [IncEncoderTimestamp_3L] -> Mux13/6
  [IncEncoderTimestamp_2R] -> Mux13/2
  [IncEncoderTimestamp_2L] -> Mux13/4
  [IncEncoderTimestamp_1L] -> Mux13/3
  [IncEncoderTimestamp_1R] -> Mux13/1
  [IncEncoderTimestamp_3R] -> Mux13/5
  Mux13/1 -> IncrementalEncoderTimestamps/1
  Data Type Conversion141/1 -> [IncEncoders_Boom]
  Mux9/1 -> AbsoluteEncoderTimestamps/1
  [HipEncoderTimestamp_3L] -> Mux9/10
  [HipEncoderTimestamp_3R] -> Mux9/9
  [MotorEncoderTimestamp_2L] -> Mux9/8
  [MotorEncoderTimestamp_1L] -> Mux9/7
  [MotorEncoderTimestamp_2R] -> Mux9/6
  [MotorEncoderTimestamp_1R] -> Mux9/5
  [LegEncoderTimestamp_2L] -> Mux9/4
  [LegEncoderTimestamp_1L] -> Mux9/3
  [LegEncoderTimestamp_2R] -> Mux9/2
  [LegEncoderTimestamp_1R] -> Mux9/1
  Mux8/1 -> MedullaID/1
  [ID_3L] -> Mux8/6
  [ID_3R] -> Mux8/3
  [ID_2R] -> Mux8/2
  [ID_1R] -> Mux8/1
  [ID_1L] -> Mux8/4
  [ID_IMU] -> Mux8/7
  [ID_2L] -> Mux8/5
  Mux12/1 -> IncrementalEncoders/1
  Mux14/1 -> AbsoluteEncoders/1
  [Thermistors_3R] -> Mux7/3
  [Thermistors_3L] -> Mux7/6
  [Thermistors_2R] -> Mux7/2
  [Thermistors_1L] -> Mux7/4
  [Thermistors_2L] -> Mux7/5
  [Thermistors_1R] -> Mux7/1
  Motor Command/1 -> Demux1/1
  ConvertThermistors/1(Temperatures) -> Temperatures/1
  Mux7/1 -> ConvertThermistors/1(adc_value)
  [HipEncoder_3L] -> Mux14/10
  [HipEncoder_3R] -> Mux14/9
  [MotorEncoder_2L] -> Mux14/8
  [MotorEncoder_1L] -> Mux14/7
  [MotorEncoder_2R] -> Mux14/6
  [MotorEncoder_1R] -> Mux14/5
  IMU Command/1 -> [IMUCommand]
  [LegEncoder_2L] -> Mux14/4
  [LegEncoder_1L] -> Mux14/3
  [LegEncoder_2R] -> Mux14/2
  [LegEncoder_1R] -> Mux14/1
  [IncEncoder_3L] -> Mux12/6
  [IncEncoder_2L] -> Mux12/4
  [IncEncoder_1L] -> Mux12/3
  [IncEncoder_3R] -> Mux12/5
  [IncEncoder_2R] -> Mux12/2
  [IncEncoder_1R] -> Mux12/1
  Data Type Conversion74/1 -> [MotorEncoder_2R]
  Data Type Conversion73/1 -> [LegEncoder_2R]
  Data Type Conversion50/1 -> [MotorEncoder_1R]
  Data Type Conversion49/1 -> [LegEncoder_1R]
  Data Type Conversion26/1 -> [MotorEncoder_2L]
  Data Type Conversion25/1 -> [LegEncoder_2L]
  Data Type Conversion1/1 -> [MotorEncoder_1L]
  Data Type Conversion3/1 -> [LegEncoder_1L]
  Data Type Conversion4/1 -> [LimitSwitch_1L]
  Data Type Conversion2/1 -> [ToeSensor_1L]
  Data Type Conversion28/1 -> [LimitSwitch_2L]
  Data Type Conversion27/1 -> [ToeSensor_2L]
  Data Type Conversion52/1 -> [LimitSwitch_1R]
  Data Type Conversion51/1 -> [ToeSensor_1R]
  Data Type Conversion75/1 -> [ToeSensor_2R]
  Data Type Conversion76/1 -> [LimitSwitch_2R]
  [ToeSensor_2L] -> Mux11/4
  [ToeSensor_1L] -> Mux11/3
  [ToeSensor_2R] -> Mux11/2
  [ToeSensor_1R] -> Mux11/1
  [LimitSwitch_3L] -> Mux1/6
  [LimitSwitch_2L] -> Mux1/5
  [LimitSwitch_1L] -> Mux1/4
  [LimitSwitch_3R] -> Mux1/3
  [LimitSwitch_2R] -> Mux1/2
  [LimitSwitch_1R] -> Mux1/1
  Data Type Conversion112/1 -> [LimitSwitch_3L]
  Data Type Conversion157/1 -> [LimitSwitch_3R]
  Demux1/5 -> [MotorCommand_3R]
  Demux1/4 -> [MotorCommand_2R]
  Demux1/3 -> [MotorCommand_1R]
  Demux1/2 -> [MotorCommand_2L]
  Demux1/1 -> [MotorCommand_1L]
  [MotorCommand_3L] -> HipMedulla_3L/3(MotorCmd)
  Demux1/6 -> [MotorCommand_3L]
  [MotorCommand_3R] -> HipMedulla_3R/3(MotorCmd)
  [MotorCommand_2R] -> LegMedulla_2R/3(MotorCmd)
  [MotorCommand_1R] -> LegMedulla_1R/3(MotorCmd)
  [MotorCommand_2L] -> LegMedulla_2L/3(MotorCmd)
  [MotorCommand_1L] -> LegMedulla_1L/3(MotorCmd)
  [MedullaCommand] -> HipMedulla_3L/1(MedullaCmd)
  [MedullaCommand] -> HipMedulla_3R/1(MedullaCmd)
  [MedullaCommand] -> LegMedulla_1L/1(MedullaCmd)
  [MedullaCommand] -> LegMedulla_2L/1(MedullaCmd)
  [MedullaCommand] -> LegMedulla_2R/1(MedullaCmd)
  [MedullaCommand] -> LegMedulla_1R/1(MedullaCmd)
  [MedullaCounter] -> LegMedulla_2L/2(MedullaCounter)
  [MedullaCounter] -> LegMedulla_1R/2(MedullaCounter)
  [MedullaCounter] -> LegMedulla_2R/2(MedullaCounter)
  [MedullaCounter] -> HipMedulla_3R/2(MedullaCounter)
  [MedullaCounter] -> HipMedulla_3L/2(MedullaCounter)
  [MedullaCounter] -> LegMedulla_1L/2(MedullaCounter)
  Counter/1 -> [MedullaCounter]
  [Counter_IMU] -> Mux10/7
  [Counter_3L] -> Mux10/6
  [Counter_2L] -> Mux10/5
  [Counter_1L] -> Mux10/4
  [Counter_3R] -> Mux10/3
  [Counter_2R] -> Mux10/2
  [Counter_1R] -> Mux10/1
  Mux10/1 -> Counters/1
  Mux6/1 -> ErrorFlags/1  "ErrorFlags"
  Mux5/1 -> MedullaState/1  "MedullaState"
  ConvertAmpCurrent/1(measuredCurrent) -> AmpMeasuredCurrent/1
  ConvertLogicVoltage/1(logicVoltage) -> LogicVoltage/1
  ConvertMotorVoltage/1(motorVoltage) -> MotorVoltage/1
  Mux4/1 -> ConvertAmpCurrent/1(adc_value)
  Mux3/1 -> ConvertLogicVoltage/1(adc_value)
  Mux2/1 -> ConvertMotorVoltage/1(adc_value)
  [State_IMU] -> Mux5/7
  [ErrorFlags_IMU] -> Mux6/7
  [ErrorFlags_3L] -> Mux6/6
  [ErrorFlags_2L] -> Mux6/5
  [ErrorFlags_1L] -> Mux6/4
  [ErrorFlags_3R] -> Mux6/3
  [ErrorFlags_2R] -> Mux6/2
  [ErrorFlags_1R] -> Mux6/1
  [State_3L] -> Mux5/6
  [State_2L] -> Mux5/5
  [State_1L] -> Mux5/4
  [State_3R] -> Mux5/3
  [State_2R] -> Mux5/2
  [State_1R] -> Mux5/1
  [AmpMeasuredCurrent_3L] -> Mux4/6
  [AmpMeasuredCurrent_2L] -> Mux4/5
  [AmpMeasuredCurrent_1L] -> Mux4/4
  [AmpMeasuredCurrent_3R] -> Mux4/3
  [AmpMeasuredCurrent_2R] -> Mux4/2
  [AmpMeasuredCurrent_1R] -> Mux4/1
  [LogicVoltage_3L] -> Mux3/6
  [LogicVoltage_2L] -> Mux3/5
  [LogicVoltage_1L] -> Mux3/4
  [LogicVoltage_3R] -> Mux3/3
  [LogicVoltage_2R] -> Mux3/2
  [LogicVoltage_1R] -> Mux3/1
  [MotorVoltage_3L] -> Mux2/6
  [MotorVoltage_2L] -> Mux2/5
  [MotorVoltage_1L] -> Mux2/4
  [MotorVoltage_3R] -> Mux2/3
  [MotorVoltage_2R] -> Mux2/2
  [MotorVoltage_1R] -> Mux2/1
  Data Type Conversion23/1 -> [KneeForce_1L]
  Data Type Conversion21/1 -> [AmpMeasuredCurrent_1L]
  Data Type Conversion15/1 -> [Thermistors_1L]
  Data Type Conversion14/1 -> [LogicVoltage_1L]
  Data Type Conversion13/1 -> [MotorVoltage_1L]
  Data Type Conversion12/1 -> [IncEncoderTimestamp_1L]
  Data Type Conversion11/1 -> [MotorEncoderTimestamp_1L]
  Data Type Conversion10/1 -> [LegEncoderTimestamp_1L]
  Data Type Conversion9/1 -> [IncEncoder_1L]
  Data Type Conversion8/1 -> [ErrorFlags_1L]
  Mux1/1 -> EncodeSwitches/1(Switches)
  HipMedulla_3L/13(AmpMeasuredCurrent) -> Data Type Conversion126/1
  HipMedulla_3L/12(Thermistors) -> Data Type Conversion117/1
  HipMedulla_3L/11(LogicVoltage) -> Data Type Conversion118/1
  HipMedulla_3L/10(MotorVoltage) -> Data Type Conversion116/1
  HipMedulla_3L/9(IncEncoderTimestamp) -> Data Type Conversion123/1
  HipMedulla_3L/8(HipEncoderTimestamp) -> Data Type Conversion124/1
  HipMedulla_3L/7(ErrorFlags) -> Data Type Conversion121/1
  HipMedulla_3L/6(Counter) -> Data Type Conversion122/1
  HipMedulla_3L/5(State) -> Data Type Conversion120/1
  HipMedulla_3L/4(ID) -> Data Type Conversion125/1
  Data Type Conversion125/1 -> [ID_3L]
  Data Type Conversion120/1 -> [State_3L]
  Data Type Conversion122/1 -> [Counter_3L]
  Data Type Conversion121/1 -> [ErrorFlags_3L]
  Data Type Conversion119/1 -> [IncEncoder_3L]
  Data Type Conversion124/1 -> [HipEncoderTimestamp_3L]
  Data Type Conversion123/1 -> [IncEncoderTimestamp_3L]
  Data Type Conversion116/1 -> [MotorVoltage_3L]
  Data Type Conversion118/1 -> [LogicVoltage_3L]
  Data Type Conversion117/1 -> [Thermistors_3L]
  Data Type Conversion126/1 -> [AmpMeasuredCurrent_3L]
  HipMedulla_3L/2(IncEncoder) -> Data Type Conversion119/1
  HipMedulla_3L/1(HipEncoder) -> Data Type Conversion114/1
  Data Type Conversion114/1 -> [HipEncoder_3L]
  HipMedulla_3L/3(LimitSwitch) -> Data Type Conversion112/1
  HipMedulla_3R/13(AmpMeasuredCurrent) -> Data Type Conversion111/1
  HipMedulla_3R/12(Thermistors) -> Data Type Conversion102/1
  HipMedulla_3R/11(LogicVoltage) -> Data Type Conversion103/1
  HipMedulla_3R/10(MotorVoltage) -> Data Type Conversion101/1
  HipMedulla_3R/9(IncEncoderTimestamp) -> Data Type Conversion108/1
  HipMedulla_3R/8(HipEncoderTimestamp) -> Data Type Conversion109/1
  HipMedulla_3R/7(ErrorFlags) -> Data Type Conversion106/1
  HipMedulla_3R/6(Counter) -> Data Type Conversion107/1
  HipMedulla_3R/5(State) -> Data Type Conversion105/1
  HipMedulla_3R/4(ID) -> Data Type Conversion110/1
  HipMedulla_3R/3(LimitSwitch) -> Data Type Conversion157/1
  HipMedulla_3R/2(IncEncoder) -> Data Type Conversion104/1
  HipMedulla_3R/1(HipEncoder) -> Data Type Conversion98/1
  Data Type Conversion98/1 -> [HipEncoder_3R]
  Data Type Conversion110/1 -> [ID_3R]
  Data Type Conversion105/1 -> [State_3R]
  Data Type Conversion107/1 -> [Counter_3R]
  Data Type Conversion106/1 -> [ErrorFlags_3R]
  Data Type Conversion104/1 -> [IncEncoder_3R]
  Data Type Conversion109/1 -> [HipEncoderTimestamp_3R]
  Data Type Conversion108/1 -> [IncEncoderTimestamp_3R]
  Data Type Conversion101/1 -> [MotorVoltage_3R]
  Data Type Conversion103/1 -> [LogicVoltage_3R]
  Data Type Conversion102/1 -> [Thermistors_3R]
  Data Type Conversion47/1 -> [KneeForce_2L]
  Data Type Conversion45/1 -> [AmpMeasuredCurrent_2L]
  Data Type Conversion39/1 -> [Thermistors_2L]
  Data Type Conversion38/1 -> [LogicVoltage_2L]
  Data Type Conversion37/1 -> [MotorVoltage_2L]
  Data Type Conversion36/1 -> [IncEncoderTimestamp_2L]
  Data Type Conversion35/1 -> [MotorEncoderTimestamp_2L]
  Data Type Conversion34/1 -> [LegEncoderTimestamp_2L]
  Data Type Conversion33/1 -> [IncEncoder_2L]
  Data Type Conversion32/1 -> [ErrorFlags_2L]
  Data Type Conversion31/1 -> [Counter_2L]
  Data Type Conversion30/1 -> [State_2L]
  Data Type Conversion29/1 -> [ID_2L]
  Data Type Conversion7/1 -> [Counter_1L]
  Data Type Conversion6/1 -> [State_1L]
  Data Type Conversion5/1 -> [ID_1L]
  LegMedulla_1R/1(LegEncoder) -> Data Type Conversion49/1
  LegMedulla_1L/1(LegEncoder) -> Data Type Conversion3/1
  LegMedulla_1R/2(MotorEncoder) -> Data Type Conversion50/1
  Data Type Conversion111/1 -> [AmpMeasuredCurrent_3R]
  Data Type Conversion95/1 -> [KneeForce_2R]
  Data Type Conversion93/1 -> [AmpMeasuredCurrent_2R]
  Data Type Conversion87/1 -> [Thermistors_2R]
  Data Type Conversion86/1 -> [LogicVoltage_2R]
  Data Type Conversion85/1 -> [MotorVoltage_2R]
  Data Type Conversion84/1 -> [IncEncoderTimestamp_2R]
  Data Type Conversion83/1 -> [MotorEncoderTimestamp_2R]
  Data Type Conversion82/1 -> [LegEncoderTimestamp_2R]
  Data Type Conversion81/1 -> [IncEncoder_2R]
  Data Type Conversion80/1 -> [ErrorFlags_2R]
  Data Type Conversion79/1 -> [Counter_2R]
  Data Type Conversion78/1 -> [State_2R]
  Data Type Conversion77/1 -> [ID_2R]
  Data Type Conversion71/1 -> [KneeForce_1R]
  Data Type Conversion69/1 -> [AmpMeasuredCurrent_1R]
  Data Type Conversion63/1 -> [Thermistors_1R]
  Data Type Conversion62/1 -> [LogicVoltage_1R]
  Data Type Conversion61/1 -> [MotorVoltage_1R]
  Data Type Conversion60/1 -> [IncEncoderTimestamp_1R]
  Data Type Conversion59/1 -> [MotorEncoderTimestamp_1R]
  Data Type Conversion58/1 -> [LegEncoderTimestamp_1R]
  Data Type Conversion57/1 -> [IncEncoder_1R]
  Data Type Conversion56/1 -> [ErrorFlags_1R]
  Data Type Conversion55/1 -> [Counter_1R]
  Data Type Conversion54/1 -> [State_1R]
  Data Type Conversion53/1 -> [ID_1R]
  LegMedulla_2R/3(ToeSensor) -> Data Type Conversion75/1
  LegMedulla_2R/2(MotorEncoder) -> Data Type Conversion74/1
  LegMedulla_2R/1(LegEncoder) -> Data Type Conversion73/1
  Counter/2 -> Terminator2/1
  Medulla Command/1 -> [MedullaCommand]
  LegMedulla_2R/17(KneeForce) -> Data Type Conversion95/1
  LegMedulla_2R/16(AmpMeasuredCurrent) -> Data Type Conversion93/1
  LegMedulla_2R/15(Thermistor0) -> Data Type Conversion87/1
  LegMedulla_2R/14(LogicVoltage) -> Data Type Conversion86/1
  LegMedulla_2R/13(MotorVoltage) -> Data Type Conversion85/1
  LegMedulla_2R/12(IncEncoderTimestamp) -> Data Type Conversion84/1
  LegMedulla_2R/11(MotorEncoderTimestamp) -> Data Type Conversion83/1
  LegMedulla_2R/10(LegEncoderTimestamp) -> Data Type Conversion82/1
  LegMedulla_2R/9(IncEncoder) -> Data Type Conversion81/1
  LegMedulla_2R/8(ErrorFlags) -> Data Type Conversion80/1
  LegMedulla_2R/7(Counter) -> Data Type Conversion79/1
  LegMedulla_2R/6(State) -> Data Type Conversion78/1
  LegMedulla_2R/5(ID) -> Data Type Conversion77/1
  LegMedulla_2R/4(LimitSwitch) -> Data Type Conversion76/1
  LegMedulla_1R/17(KneeForce) -> Data Type Conversion71/1
  LegMedulla_1R/16(AmpMeasuredCurrent) -> Data Type Conversion69/1
  LegMedulla_1R/15(Thermistors) -> Data Type Conversion63/1
  LegMedulla_1R/14(LogicVoltage) -> Data Type Conversion62/1
  LegMedulla_1R/13(MotorVoltage) -> Data Type Conversion61/1
  LegMedulla_1R/12(IncEncoderTimestamp) -> Data Type Conversion60/1
  LegMedulla_1R/11(MotorEncoderTimestamp) -> Data Type Conversion59/1
  LegMedulla_1R/10(LegEncoderTimestamp) -> Data Type Conversion58/1
  LegMedulla_1R/9(IncEncoder) -> Data Type Conversion57/1
  LegMedulla_1R/8(ErrorFlags) -> Data Type Conversion56/1
  LegMedulla_1R/7(Counter) -> Data Type Conversion55/1
  LegMedulla_1R/6(State) -> Data Type Conversion54/1
  LegMedulla_1R/5(ID) -> Data Type Conversion53/1
  LegMedulla_1R/4(LimitSwitch) -> Data Type Conversion52/1
  LegMedulla_1R/3(ToeSensor) -> Data Type Conversion51/1
  LegMedulla_2L/17(KneeForce) -> Data Type Conversion47/1
  LegMedulla_2L/16(AmpMeasuredCurrent) -> Data Type Conversion45/1
  LegMedulla_2L/15(Thermistors) -> Data Type Conversion39/1
  LegMedulla_2L/14(LogicVoltage) -> Data Type Conversion38/1
  LegMedulla_2L/13(MotorVoltage) -> Data Type Conversion37/1
  LegMedulla_2L/12(IncEncoderTimestamp) -> Data Type Conversion36/1
  LegMedulla_2L/11(MotorEncoderTimestamp) -> Data Type Conversion35/1
  LegMedulla_2L/10(LegEncoderTimestamp) -> Data Type Conversion34/1
  LegMedulla_2L/9(IncEncoder) -> Data Type Conversion33/1
  LegMedulla_2L/8(ErrorFlags) -> Data Type Conversion32/1
  LegMedulla_2L/7(Counter) -> Data Type Conversion31/1
  LegMedulla_2L/6(State) -> Data Type Conversion30/1
  LegMedulla_2L/5(ID) -> Data Type Conversion29/1
  LegMedulla_2L/4(LimitSwitch) -> Data Type Conversion28/1
  LegMedulla_2L/3(ToeSensor) -> Data Type Conversion27/1
  LegMedulla_2L/2(MotorEncoder) -> Data Type Conversion26/1
  LegMedulla_2L/1(LegEncoder) -> Data Type Conversion25/1
  LegMedulla_1L/17(KneeForce) -> Data Type Conversion23/1
  LegMedulla_1L/16(AmpMeasuredCurrent) -> Data Type Conversion21/1
  LegMedulla_1L/15(Thermistors) -> Data Type Conversion15/1
  LegMedulla_1L/14(LogicVoltage) -> Data Type Conversion14/1
  LegMedulla_1L/13(MotorVoltage) -> Data Type Conversion13/1
  LegMedulla_1L/12(IncEncoderTimestamp) -> Data Type Conversion12/1
  LegMedulla_1L/11(MotorEncoderTimestamp) -> Data Type Conversion11/1
  LegMedulla_1L/10(LegEncoderTimestamp) -> Data Type Conversion10/1
  LegMedulla_1L/9(IncEncoder) -> Data Type Conversion9/1
  LegMedulla_1L/8(ErrorFlags) -> Data Type Conversion8/1
  LegMedulla_1L/7(Counter) -> Data Type Conversion7/1
  LegMedulla_1L/6(State) -> Data Type Conversion6/1
  LegMedulla_1L/5(ID) -> Data Type Conversion5/1
  LegMedulla_1L/4(LimitSwitch) -> Data Type Conversion4/1
  LegMedulla_1L/3(ToeSensor) -> Data Type Conversion2/1
  LegMedulla_1L/2(MotorEncoder) -> Data Type Conversion1/1
  EncodeSwitches/1(LimitSwitchesEncoded) -> LimitSwitches/1
  Mux11/1 -> ToeSwitches/1
  "EtherCAT Init "/1 -> Data Type Conversion97/1
  Data Type Conversion97/1 -> EtherCATStatus/1
  [IMUCommand] -> Terminator5/1
  IMU_Medulla/9(Sequence) -> Data Type Conversion24/1
  IMU_Medulla/1(AngularRate) -> Data Type Conversion20/1
  IMU_Medulla/6(ErrorFlags) -> Data Type Conversion19/1
  IMU_Medulla/2(Acceleration) -> Data Type Conversion22/1
  Constant/1 -> IMU_Medulla/1(MedullaCmd)
  [MedullaCounter] -> IMU_Medulla/2(MedullaCounter)
  IMU_Medulla/3(ID) -> Data Type Conversion16/1
  IMU_Medulla/4(State) -> Data Type Conversion17/1
  IMU_Medulla/5(Counter) -> Data Type Conversion18/1
  IMU_Medulla/8(Temperature) -> Terminator6/1
  IMU_Medulla/7(CRC) -> Terminator7/1
  Data Type Conversion24/1 -> Terminator4/1, Scope 1/1, IMU Sequence/1
  Data Type Conversion20/1 -> Scope 2/1, AngularRate/1
